simulink library "Dampers_Axle1_None"  (R2026a)
settings: Solver=VariableStepAuto
libraries: fl_lib x2
Description:
  | Component of Simscape Vehicle Templates Library
  | 
  | Copyright 2018-2026 The MathWorks, Inc.
settings Model: Creator=smiller  LastModifiedBy=smiller

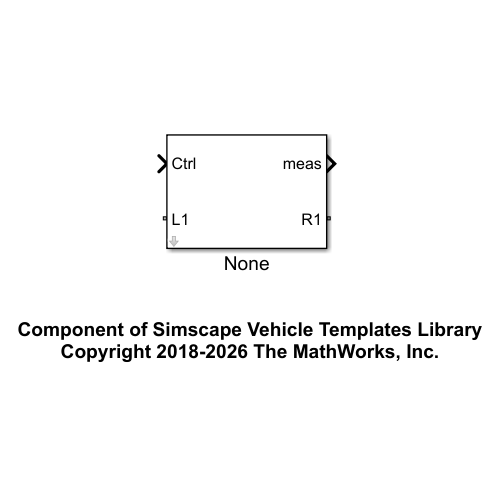
[thumbnail: Simulink's stored preview of the top-level diagram]
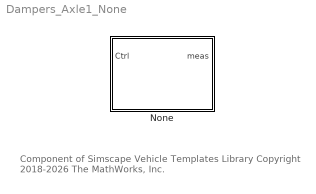
== system Dampers_Axle1_None ==
  note: Component of Simscape Vehicle Templates Library
      | Copyright 2018-2026 The MathWorks, Inc.
  None : Subsystem  VariantControl=Independent  mask(Damper System Placeholder){}
      mask help: Empty subsystem, used as a variant that omits dampers.

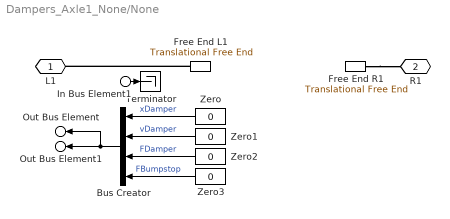
== system Dampers_Axle1_None/None ==
  In Bus Element1 : Inport  PortName=Ctrl  Element=L1
  Bus Creator : BusCreator  Inputs=4
  Free End L1 : fl_lib/Mechanical/Translational Elements/Translational Free End  v_specify=off  v_priority=None  v=0 m/s  v_nominal_specify=off  v_nominal_value=1  v_nominal_unit=m/s
  Free End R1 : fl_lib/Mechanical/Translational Elements/Translational Free End  v_specify=off  v_priority=None  v=0 m/s  v_nominal_specify=off  v_nominal_value=1  v_nominal_unit=m/s
  Terminator : Terminator
  Zero{,1..3} (4 alike) : Constant  Value=0  OutDataTypeStr=Inherit: Inherit via back propagation
  L1 : PMIOPort  Side=Left
  R1 : PMIOPort  Port=2  Side=Right
  Out Bus Element : Outport  VectorParamsAs1DForOutWhenUnconnected=off  PortName=meas  Element=L1
  Out Bus Element1 : Outport  VectorParamsAs1DForOutWhenUnconnected=off  PortName=meas  Element=R1
  wires:
  Bus Creator/1 -> Out Bus Element/1, Out Bus Element1/1
  In Bus Element1/1 -> Terminator/1
  Zero/1 -> Bus Creator/1  "xDamper"
  Zero1/1 -> Bus Creator/2  "vDamper"
  Zero2/1 -> Bus Creator/3  "FDamper"
  Zero3/1 -> Bus Creator/4  "FBumpstop"
  connections:
  Free End L1/LConn1 -- L1/RConn1
  Free End R1/LConn1 -- R1/RConn1
